simulink model "helikopter"  (R2014a)
settings: Solver=ode1  StartTime=0.0  StopTime=inf  FixedStep=0.002  RelTol=1e-3
PostLoadFcn:
  | qc_set_target_type(getConfigSet(bdroot, 'QUARC Default Target Configuration'));
values from neighbouring files (symbols this model uses):
  K_ed = 8    [init02.m]    (also in init03.m = 10; init04.m = 5.5; init05.m = 10; init06.m = 10)
  K_ei = 2.5    [init02.m]    (also in init03.m = 4; init04.m = 4; init05.m = 3.3; init06.m = 3.3)
  K_ep = 10    [init02.m]    (also in init03.m = 9; init04.m = 7; init05.m = 9; init06.m = 7)
  K_pd = w_c/K_1    (= 3.53504587156)    [init02.m]    (also in init03.m = 3.08816258919; init04.m = 3.74170380079; init05.m = 3.69819571865; init06.m = 4.04246797256)
  K_pp = (sqrt(2)*w_c^2)/K_1    [init02.m]    (also in init03.m; init04.m; init05.m; init06.m)
  KalibElevasjon = -.105    (= -0.105)    [init02.m]    (also in init03.m = -0.1055; init04.m; init05.m; init06.m = -0.0925)
  KalibPitch = .0879    (= 0.0879)    [init02.m]    (also in init03.m; init04.m; init05.m; init06.m = 0.08785)
  KalibVandring = .0879/2    (= 0.04395)    [init02.m]    (also in init03.m; init04.m = 0.044; init05.m = 0.043975; init06.m = 0.044)
  V_b_eq = .6    (= 0.6)    [init02.m]    (also in init03.m; init04.m = 0.691; init05.m = 0.615; init06.m = 0.58)
  V_f_eq = .635    (= 0.635)    [init02.m]    (also in init03.m = 0.625; init04.m = 0.595; init05.m = 0.63; init06.m = 0.6)
undefined symbols (not defined in the file or in its folder): HIL
libraries: quarc_library x3
settings Model: SimulationMode=external  ExtModeTrigDuration=5000  Creator=Rchan  LastModifiedBy=knutgb
settings SolverCC: PositivePriorityOrder=on
settings DataIOCC: SignalLoggingSaveFormat=ModelDataLogs
settings OptimizationCC: ExpressionDepthLimit=2147483647  InitFltsAndDblsToZero=on
settings DebuggingCC: SaveWithParameterizedLinksMsg=none  UnderspecifiedInitializationDetection=Classic  MultiTaskDSMMsg=warning  MultiTaskCondExecSysMsg=none  FcnCallInpInsideContextMsg=UseLocalSettings  StateNameClashWarn=warning
settings RTWCC: SystemTargetFile=quarc_win64.tlc  TemplateMakefile=quarc_default_tmf  Description=QUARC Win64 Target  ProcessScript=quarc_win64_make_rtw_hook
settings STFCustomTargetCC: CPPClassGenCompliant=on
settings GRTTargetCC: ParMdlRefBuildCompliant=off  CompOptLevelCompliant=off  CombineOutputUpdateFcns=off  MatFileLogging=off  GRTInterface=on  ExtMode=on  ExtModeMexFile=quarc_comm

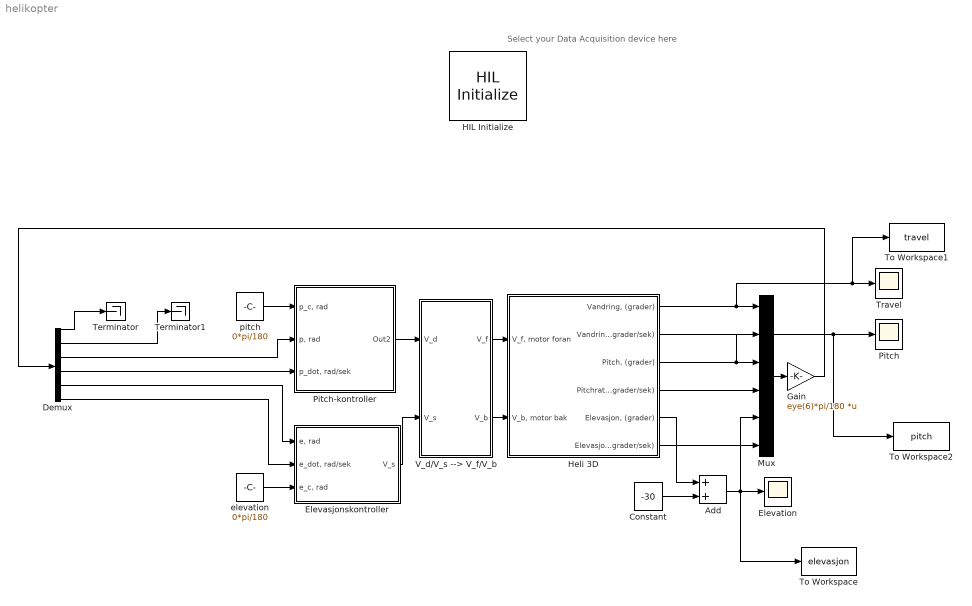
== system helikopter ==
  note: Select your Data Acquisition device here
  Add : Sum
  Constant : Constant  Value=-30
  Demux : Demux  Outputs=6
  Elevasjonskontroller : Subsystem
  Elevation : Scope
      settings: TimeRange=10  YMin=1.5  YMax=2.2
  Gain : Gain  Gain=eye(6)*pi/180  Multiplication=Matrix(K*u)
  HIL Initialize : quarc_library/Data Acquisition/Generic/Configuration/HIL Initialize  Priority=-99  object_name=HIL-1  board_type=q8_usb  board_number=0  board_options=update_rate=normal;decimation=1  exclusive=off  active=off  hardware_clocks=[0:2]  clock_modes=[]  initial_clock_frequencies=[]  set_clock_params_at_start=off  set_clock_params_at_switch_in=off  set_clock_frequencies_at_start=off  set_clock_frequencies_at_switch_in=off  analog_input_channels=[0:7]  analog_input_maximums=10  analog_input_minimums=-10  set_analog_input_params_at_start=on  set_analog_input_params_at_switch_in=off  analog_output_channels=[0:7]  analog_output_maximums=10  analog_output_minimums=-10  initial_analog_outputs=[0]  final_analog_outputs=[0]  watchdog_analog_outputs=0  set_analog_output_params_at_start=on  set_analog_output_params_at_switch_in=off  set_analog_outputs_at_start=on  set_analog_outputs_at_switch_in=off  set_analog_outputs_at_terminate=on  set_analog_outputs_at_switch_out=off  set_analog_outputs_on_watchdog=off  digital_input_channels=[]  digital_output_channels=[]  digital_output_configuration=[]  initial_digital_outputs=[1]  final_digital_outputs=[1]  watchdog_digital_outputs=[1]  set_digital_output_params_at_start=off  set_digital_output_params_at_switch_in=off  set_digital_outputs_at_start=on  set_digital_outputs_at_switch_in=off  set_digital_outputs_at_terminate=on  set_digital_outputs_at_switch_out=off  set_digital_outputs_on_watchdog=off  encoder_channels=[0:7]  quadrature=[4]  encoder_filter_frequency=[]  initial_encoder_counts=[0]  set_encoder_params_at_start=on  set_encoder_params_at_switch_in=off  set_encoder_counts_at_start=on  set_encoder_counts_at_switch_in=off  pwm_channels=[0:7]  pwm_modes=0  pwm_frequency=99.532799999999995e6/4095  pwm_configuration=[0]  pwm_alignment=[0]  pwm_polarity=[1]  pwm_leading_deadband=[0]  pwm_trailing_deadband=[0]  initial_pwm_outputs=[0]  final_pwm_outputs=[0]  watchdog_pwm_outputs=[0]  set_pwm_params_at_start=on  set_pwm_params_at_switch_in=off  set_pwm_outputs_at_start=on  set_pwm_outputs_at_switch_in=off  set_pwm_outputs_at_terminate=on  set_pwm_outputs_at_switch_out=off  set_pwm_outputs_on_watchdog=off  other_output_channels=[]  initial_other_outputs=[]  final_other_outputs=[]  watchdog_other_outputs=[]  set_other_outputs_at_start=off  set_other_outputs_at_switch_in=off  set_other_outputs_at_terminate=off  set_other_outputs_at_switch_out=off  set_other_outputs_on_watchdog=off
  Heli 3D : Subsystem
  Mux : Mux  Inputs=6
  Pitch : Scope
      settings: TimeRange=10  YMin=-15  YMax=95  SaveName=ScopeData2
  Pitch-kontroller : Subsystem
  Terminator : Terminator
  Terminator1 : Terminator
  To Workspace : ToWorkspace  VariableName=elevasjon  SaveFormat=Structure With Time  SampleTime=-1
  To Workspace1 : ToWorkspace  VariableName=travel  SaveFormat=Structure With Time  SampleTime=-1
  To Workspace2 : ToWorkspace  VariableName=pitch  SaveFormat=Structure With Time  SampleTime=-1
  Travel : Scope
      settings: YMin=-375  YMax=25  SaveName=ScopeData3
  V_d/V_s --> V_f/V_b : Subsystem
  elevation : Constant  Value=0*pi/180
  pitch : Constant  Value=0*pi/180
  wires:
  Pitch-kontroller/1(Out2) -> V_d/V_s --> V_f/V_b/1(V_d)
  Elevasjonskontroller/1(V_s) -> V_d/V_s --> V_f/V_b/2(V_s)
  Heli 3D/1("Vandring, (grader)") -> Mux/1, Travel/1, To Workspace1/1
  Heli 3D/4("Pitchrate, (grader/sek)") -> Mux/4
  Heli 3D/5("Elevasjon, (grader)") -> Add/1
  Heli 3D/6(Elevasjonsrate (grader/sek)) -> Mux/6
  Mux/1 -> Gain/1
  Demux/1 -> Terminator/1
  Demux/2 -> Terminator1/1
  Gain/1 -> Demux/1
  pitch/1 -> Pitch-kontroller/1("p_c, rad")
  Demux/3 -> Pitch-kontroller/2("p, rad")
  Demux/4 -> Pitch-kontroller/3("p_dot, rad/sek")
  Demux/5 -> Elevasjonskontroller/1("e, rad")
  Demux/6 -> Elevasjonskontroller/2("e_dot, rad/sek")
  elevation/1 -> Elevasjonskontroller/3("e_c, rad")
  Constant/1 -> Add/2
  Add/1 -> Elevation/1, Mux/5, To Workspace/1
  Heli 3D/3("Pitch, (grader)") -> Mux/3, To Workspace2/1, Pitch/1
  Heli 3D/2("Vandringsrate, (grader/sek)") -> Mux/2
  V_d/V_s --> V_f/V_b/1(V_f) -> Heli 3D/1("V_f, motor foran")
  V_d/V_s --> V_f/V_b/2(V_b) -> Heli 3D/2("V_b, motor bak")

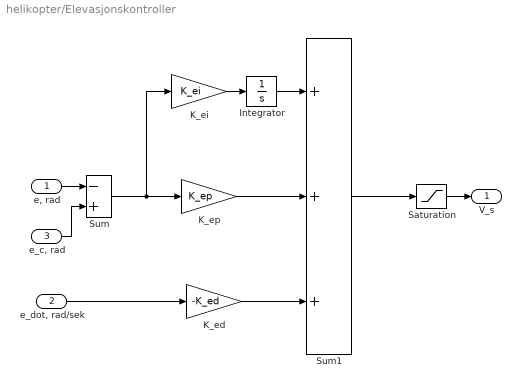
== system helikopter/Elevasjonskontroller ==
  "e, rad" : Inport
  "e_dot, rad/sek" : Inport  Port=2
  "e_c, rad" : Inport  Port=3
  Integrator : Integrator  LimitOutput=on
  K_ed : Gain  Gain=-K_ed  SaturateOnIntegerOverflow=on  OutDataTypeStr=Inherit: Same as input  ParamDataTypeStr=Inherit: Same as input
  K_ei : Gain  Gain=K_ei  SaturateOnIntegerOverflow=on  OutDataTypeStr=Inherit: Same as input  ParamDataTypeStr=Inherit: Same as input
  K_ep : Gain  Gain=K_ep  SaturateOnIntegerOverflow=on  OutDataTypeStr=Inherit: Same as input  ParamDataTypeStr=Inherit: Same as input
  Saturation : Saturate  UpperLimit=10  LowerLimit=-10
  Sum : Sum  Inputs=-+  SaturateOnIntegerOverflow=on  InputSameDT=on  OutDataTypeStr=Inherit: Same as first input
  Sum1 : Sum  Inputs=+++  SaturateOnIntegerOverflow=on  InputSameDT=on  OutDataTypeStr=Inherit: Same as first input
  V_s : Outport  InitialOutput=0
  wires:
  Sum/1 -> K_ei/1, K_ep/1
  "e, rad"/1 -> Sum/1
  "e_c, rad"/1 -> Sum/2
  "e_dot, rad/sek"/1 -> K_ed/1
  Saturation/1 -> V_s/1
  Sum1/1 -> Saturation/1
  K_ep/1 -> Sum1/2
  K_ed/1 -> Sum1/3
  Integrator/1 -> Sum1/1
  K_ei/1 -> Integrator/1

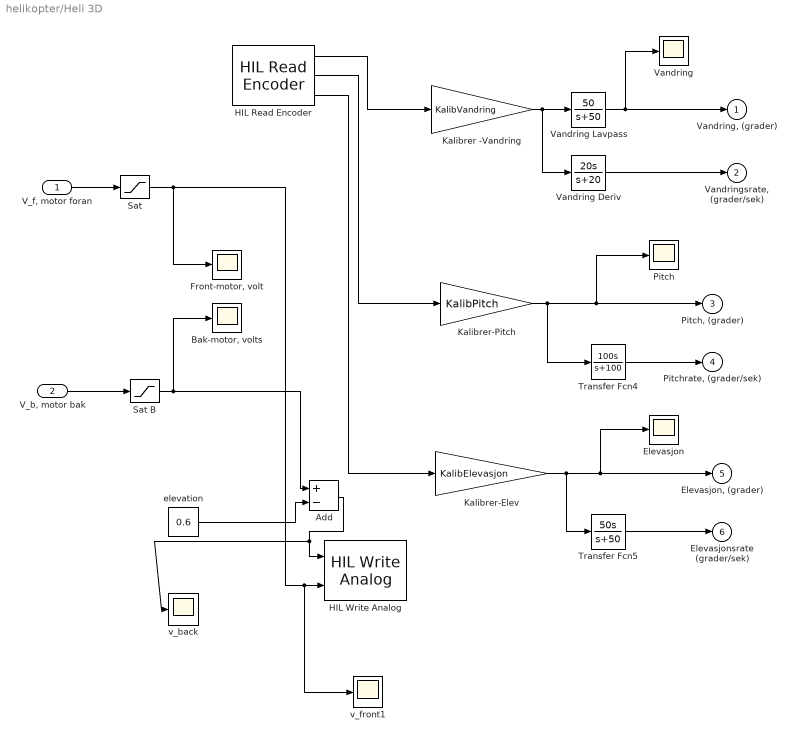
== system helikopter/Heli 3D ==
  "V_f, motor foran" : Inport
  "V_b, motor bak" : Inport  Port=2
  Add : Sum  Inputs=+-
  "Bak-motor, volts" : Scope
      settings: TickLabels=on  TimeRange=1.234000  YMin=-1.560000  YMax=1.560000
  Elevasjon : Scope
      settings: TickLabels=on  TimeRange=1.234000  YMin=-1.56  YMax=1.56
  "Front-motor, volt" : Scope
      settings: TickLabels=on  TimeRange=1.234000  YMin=-1.560000  YMax=1.560000
  HIL Read Encoder : quarc_library/Data Acquisition/Generic/Immediate I//O/HIL Read Encoder  object_name=HIL-1  channels=[0,1,2]  sample_time=qc_get_step_size  active=on  vector_output=off  data_type_mode=Inherit via back propagation  data_type=double
  HIL Write Analog : quarc_library/Data Acquisition/Generic/Immediate I//O/HIL Write Analog  object_name=HIL-1  channels=[1,0]  sample_time=-1  active=off  vector_input=off
  Kalibrer -Vandring : Gain  Gain=KalibVandring  SaturateOnIntegerOverflow=on  OutDataTypeStr=Inherit: Same as input  ParamDataTypeStr=Inherit: Same as input
  Kalibrer-Elev : Gain  Gain=KalibElevasjon  SaturateOnIntegerOverflow=on  OutDataTypeStr=Inherit: Same as input  ParamDataTypeStr=Inherit: Same as input
  Kalibrer-Pitch : Gain  Gain=KalibPitch  SaturateOnIntegerOverflow=on  OutDataTypeStr=Inherit: Same as input  ParamDataTypeStr=Inherit: Same as input
  Pitch : Scope
      settings: TickLabels=on  TimeRange=1.000000  YMin=-1  YMax=1
  Sat : Saturate  UpperLimit=5  LowerLimit=-5
  Sat B : Saturate  UpperLimit=5  LowerLimit=-5
  Transfer Fcn4 : TransferFcn  Numerator=[100 0]  Denominator=[1 100]
  Transfer Fcn5 : TransferFcn  Numerator=[50 0]  Denominator=[1 50]
  Vandring : Scope
      settings: TickLabels=on  TimeRange=1.000000  YMin=-1.000000  YMax=1.000000
  Vandring Deriv : TransferFcn  Numerator=[20 0]  Denominator=[1 20]
  Vandring Lavpass : TransferFcn  Numerator=[50]  Denominator=[1 50]
  elevation : Constant  Value=0.6
  v_back : Scope
      settings: TimeRange=10  YMin=1.1  YMax=2.4  SaveName=ScopeData7
  v_front1 : Scope
      settings: TimeRange=10  YMin=1.1  YMax=2.4  SaveName=ScopeData6
  "Vandring, (grader)" : Outport  InitialOutput=0
  "Vandringsrate, (grader/sek)" : Outport  Port=2  InitialOutput=0
  "Pitch, (grader)" : Outport  Port=3  InitialOutput=0
  "Pitchrate, (grader/sek)" : Outport  Port=4  InitialOutput=0
  "Elevasjon, (grader)" : Outport  Port=5  InitialOutput=0
  Elevasjonsrate (grader/sek) : Outport  Port=6  InitialOutput=0
  wires:
  Vandring Deriv/1 -> "Vandringsrate, (grader/sek)"/1
  Vandring Lavpass/1 -> Vandring/1, "Vandring, (grader)"/1
  Kalibrer -Vandring/1 -> Vandring Deriv/1, Vandring Lavpass/1
  Kalibrer-Pitch/1 -> Pitch/1, "Pitch, (grader)"/1, Transfer Fcn4/1
  Transfer Fcn4/1 -> "Pitchrate, (grader/sek)"/1
  Kalibrer-Elev/1 -> Transfer Fcn5/1, Elevasjon/1, "Elevasjon, (grader)"/1
  Transfer Fcn5/1 -> Elevasjonsrate (grader/sek)/1
  Sat/1 -> "Front-motor, volt"/1, HIL Write Analog/2, v_front1/1
  Sat B/1 -> "Bak-motor, volts"/1, Add/1
  "V_f, motor foran"/1 -> Sat/1
  "V_b, motor bak"/1 -> Sat B/1
  HIL Read Encoder/1 -> Kalibrer -Vandring/1
  HIL Read Encoder/2 -> Kalibrer-Pitch/1
  HIL Read Encoder/3 -> Kalibrer-Elev/1
  elevation/1 -> Add/2
  Add/1 -> HIL Write Analog/1, v_back/1

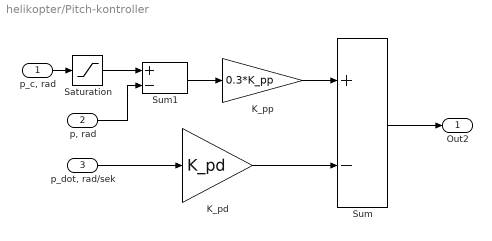
== system helikopter/Pitch-kontroller ==
  "p_c, rad" : Inport
  "p, rad" : Inport  Port=2
  "p_dot, rad/sek" : Inport  Port=3
  K_pd : Gain  Gain=K_pd  SaturateOnIntegerOverflow=on  OutDataTypeStr=Inherit: Same as input  ParamDataTypeStr=Inherit: Same as input
  K_pp : Gain  Gain=0.3*K_pp  SaturateOnIntegerOverflow=on  OutDataTypeStr=Inherit: Same as input  ParamDataTypeStr=Inherit: Same as input
  Saturation : Saturate  UpperLimit=50*pi/180  LowerLimit=-50*pi/180
  Sum : Sum  Inputs=+-  SaturateOnIntegerOverflow=on  InputSameDT=on  OutDataTypeStr=Inherit: Same as first input
  Sum1 : Sum  Inputs=+-  SaturateOnIntegerOverflow=on  InputSameDT=on  OutDataTypeStr=Inherit: Same as first input
  Out2 : Outport  InitialOutput=0
  wires:
  Saturation/1 -> Sum1/1
  "p_c, rad"/1 -> Saturation/1
  Sum1/1 -> K_pp/1
  Sum/1 -> Out2/1
  K_pp/1 -> Sum/1
  K_pd/1 -> Sum/2
  "p_dot, rad/sek"/1 -> K_pd/1
  "p, rad"/1 -> Sum1/2

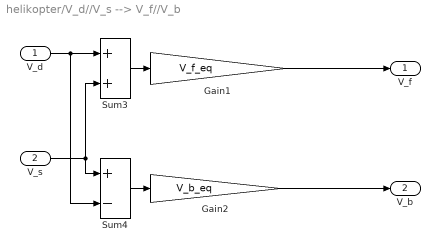
== system helikopter/V_d//V_s --> V_f//V_b ==
  V_d : Inport
  V_s : Inport  Port=2
  Gain1 : Gain  Gain=V_f_eq  SaturateOnIntegerOverflow=on  OutDataTypeStr=Inherit: Same as input  ParamDataTypeStr=Inherit: Same as input
  Gain2 : Gain  Gain=V_b_eq  SaturateOnIntegerOverflow=on  OutDataTypeStr=Inherit: Same as input  ParamDataTypeStr=Inherit: Same as input
  Sum3 : Sum  SaturateOnIntegerOverflow=on  InputSameDT=on  OutDataTypeStr=Inherit: Same as first input
  Sum4 : Sum  Inputs=+-  SaturateOnIntegerOverflow=on  InputSameDT=on  OutDataTypeStr=Inherit: Same as first input
  V_f : Outport  InitialOutput=0
  V_b : Outport  Port=2  InitialOutput=0
  wires:
  Gain2/1 -> V_b/1
  Gain1/1 -> V_f/1
  V_d/1 -> Sum4/2, Sum3/1
  Sum4/1 -> Gain2/1
  Sum3/1 -> Gain1/1
  V_s/1 -> Sum3/2, Sum4/1
